simulink model "inv"  (R2024b)
settings: Solver=VariableStepAuto  StartTime=0.0  StopTime=0.5  RelTol=1e-3
InitFcn:
  | systemIni
values from neighbouring files (symbols this model uses):
  omega = 1    [systemIni.m]
  PWMrat = 39    [systemIni.m]
  Tc = 10e-6    (= 1e-05)    [systemIni.m]
  Ts = 1e-6    (= 1e-06)    [systemIni.m]
  v_ref = Vdc    [systemIni.m]
  Vdc = 550/Vb    [systemIni.m]
  w_b = wb    [systemIni.m]
libraries: spspowerguiLib x2
settings Model: Creator=PetrosK  LastModifiedBy=horak
settings DebuggingCC: UnderspecifiedInitializationDetection=Classic  MergeDetectMultiDrivingBlocksExec=none
settings ModelReferenceCC: PropagateSignalLabelsOutOfModel=off

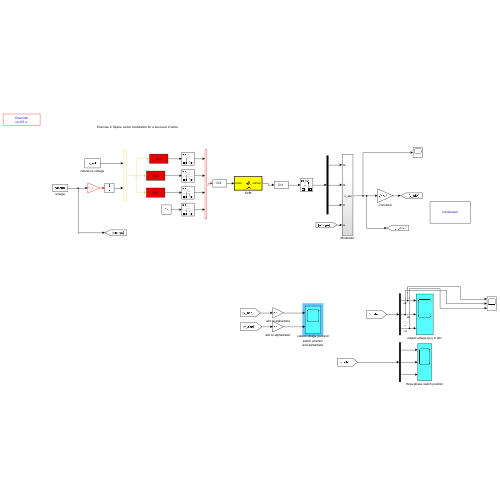
[thumbnail: Simulink's stored preview of the top-level diagram]
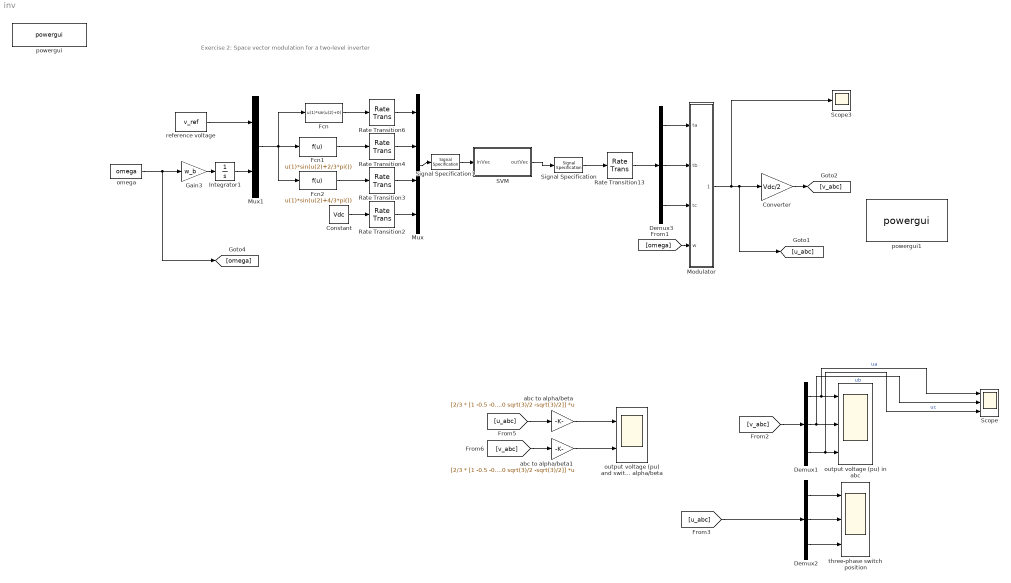
== system inv ==
  note: Exercise 2: Space vector modulation for a two-level inverter
  Constant : Constant  Value=Vdc  VectorParams1D=off
  Converter : Gain  Gain=Vdc/2  SaturateOnIntegerOverflow=on  OutDataTypeStr=Inherit: Same as input  ParamDataTypeStr=Inherit: Same as input
  Demux1 : Demux  Outputs=3
  Demux2 : Demux  Outputs=3
  Demux3 : Demux  Outputs=3
  Fcn : Fcn  Expr=u(1)*sin(u(2)+0)
  Fcn1 : Fcn  Expr=u(1)*sin(u(2)+2/3*pi())
  Fcn2 : Fcn  Expr=u(1)*sin(u(2)+4/3*pi())
  Gain3 : Gain  Gain=w_b
  Integrator1 : Integrator
  Modulator : Subsystem
  Mux : Mux
  Mux1 : Mux  Inputs=2
  Rate Transition13 : RateTransition  Deterministic=off  OutPortSampleTime=Ts
  Rate Transition{2..4,6} (4 alike) : RateTransition  Deterministic=off  OutPortSampleTime=Tc
  SVM : MATLAB Function  TreatAsAtomicUnit=on
  Scope : Scope  NumInputPorts=3
  Scope3 : Scope
  Signal Specification : SignalSpecification  Dimensions=3
  Signal Specification1 : SignalSpecification  Dimensions=4
  abc to alpha/beta : Gain  Gain=[2/3 * [1 -0.5 -0.5;0 sqrt(3)/2 -sqrt(3)/2]]  Multiplication=Matrix(K*u)  SaturateOnIntegerOverflow=on  OutDataTypeStr=Inherit: Same as input  ParamDataTypeStr=Inherit: Same as input
  abc to alpha/beta1 : Gain  Gain=[2/3 * [1 -0.5 -0.5;0 sqrt(3)/2 -sqrt(3)/2]]  Multiplication=Matrix(K*u)  SaturateOnIntegerOverflow=on  OutDataTypeStr=Inherit: Same as input  ParamDataTypeStr=Inherit: Same as input
  omega : Constant  Value=omega  VectorParams1D=off
  output voltage (pu) and switch position and alpha/beta : Scope  NumInputPorts=2
  output voltage (pu) in abc : Scope  NumInputPorts=3
  powergui : spspowerguiLib/powergui  Priority=1  SimulationMode=Discrete  SampleTime=Tc  frequency=60  Iterations=50  frequencyindice=0  Pbase=100e6  ErrMax=1e-4  UnitsV=kV  UnitsW=MW  buscounter=0  FunctionMessages=off  echomessages=off  EnableUseOfTLC=off  CurrentSourceSwitches=off  DisableSnubberDevices=off  DisableRonSwitches=off  DisableVfSwitches=off  DisplayEquations=off  AutomaticDiscreteSolvers=off  SolverType=Tustin  Interpol=off  ExternalGateDelay=off  methode=off  Ts=0  x0status=zero  SPID=off  SwTol=0  HookPort=off  NonlinearTolerance=1e-4  nMaxIteration=100  ContinueOnMaxIteration=off  RestoreLinks=warning  ResistiveCurrentMeasurement=off  Frange=[0:2:500]  Ylog=off  Xlog=on  ShowGrid=off  save=off  variable=ZData  structure=u_alpha  ZoomFFT=off  StartTime=0.02  cycles=1  DisplayStyle=1  fundamental=50  FreqAxis=off  MaxFrequency=4000  frequencyindicesteady=1  RmsSteady=1  display=off
  powergui1 : spspowerguiLib/powergui  Priority=1  SimulationMode=Continuous  SampleTime=50e-6  frequency=60  Iterations=50  frequencyindice=60  Pbase=100e6  ErrMax=1e-4  UnitsV=kV  UnitsW=MW  buscounter=0  FunctionMessages=off  echomessages=on  EnableUseOfTLC=off  CurrentSourceSwitches=off  DisableSnubberDevices=off  DisableRonSwitches=off  DisableVfSwitches=off  DisplayEquations=off  AutomaticDiscreteSolvers=off  SolverType=Tustin/Backward Euler (TBE)  Interpol=off  ExternalGateDelay=off  methode=off  Ts=100  x0status=blocks  SPID=on  SwTol=0  HookPort=off  NonlinearTolerance=1e-4  nMaxIteration=100  ContinueOnMaxIteration=off  RestoreLinks=warning  ResistiveCurrentMeasurement=off  Frange=[0:2:500]  Ylog=off  Xlog=on  ShowGrid=off  save=off  variable=ZData  structure=0  ZoomFFT=off  StartTime=0.0  cycles=1  DisplayStyle=1  fundamental=60  FreqAxis=off  MaxFrequency=1000  frequencyindicesteady=1  RmsSteady=1  display=off
  reference voltage : Constant  Value=v_ref  VectorParams1D=off
  three-phase switch position : Scope  NumInputPorts=3
  wires:
  SVM/1(outVec) -> Signal Specification/1
  Demux3/2 -> Modulator/2(tb)
  Demux3/3 -> Modulator/3(tc)
  Demux3/1 -> Modulator/1(ta)
  Constant/1 -> Rate Transition2/1
  Rate Transition13/1 -> Demux3/1
  Signal Specification1/1 -> SVM/1(inVec)
  Signal Specification/1 -> Rate Transition13/1
  Mux/1 -> Signal Specification1/1
  Rate Transition2/1 -> Mux/4
  Rate Transition3/1 -> Mux/3
  Rate Transition4/1 -> Mux/2
  Rate Transition6/1 -> Mux/1
  Fcn/1 -> Rate Transition6/1
  Fcn1/1 -> Rate Transition4/1
  Fcn2/1 -> Rate Transition3/1
  Mux1/1 -> Fcn2/1, Fcn1/1, Fcn/1
  [omega] -> Modulator/4(w)
  reference voltage/1 -> Mux1/1
  Gain3/1 -> Integrator1/1
  Integrator1/1 -> Mux1/2
  Demux1/2 -> Scope/2, output voltage (pu) in abc/2  "ub"
  Demux1/3 -> Scope/3, output voltage (pu) in abc/3  "uc"
  abc to alpha/beta/1 -> output voltage (pu) and switch position and alpha/beta/1
  [v_abc] -> Demux1/1
  abc to alpha/beta1/1 -> output voltage (pu) and switch position and alpha/beta/2
  [u_abc] -> abc to alpha/beta/1
  [v_abc] -> abc to alpha/beta1/1
  Modulator/1(u_abc) -> Scope3/1, [u_abc], Converter/1
  omega/1 -> [omega], Gain3/1
  Demux1/1 -> Scope/1, output voltage (pu) in abc/1  "ua"
  Demux2/2 -> three-phase switch position/2
  [u_abc] -> Demux2/1
  Demux2/1 -> three-phase switch position/1
  Demux2/3 -> three-phase switch position/3
  Converter/1 -> [v_abc]

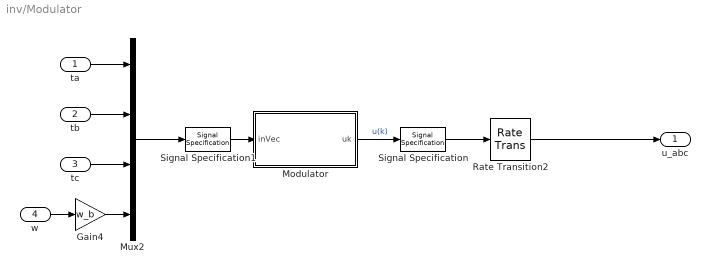
== system inv/Modulator ==
  ta : Inport
  tb : Inport  Port=2
  tc : Inport  Port=3
  w : Inport  Port=4
  Gain4 : Gain  Gain=w_b
  Modulator : MATLAB Function  TreatAsAtomicUnit=on
  Mux2 : Mux
  Rate Transition2 : RateTransition  OutPortSampleTime=Ts
  Signal Specification : SignalSpecification  Dimensions=3
  Signal Specification1 : SignalSpecification  Dimensions=4
  u_abc : Outport
  wires:
  ta/1 -> Mux2/1
  tb/1 -> Mux2/2
  tc/1 -> Mux2/3
  Modulator/1(uk) -> Signal Specification/1  "u(k)"
  Signal Specification/1 -> Rate Transition2/1
  Rate Transition2/1 -> u_abc/1
  Mux2/1 -> Signal Specification1/1
  w/1 -> Gain4/1
  Signal Specification1/1 -> Modulator/1(inVec)
  Gain4/1 -> Mux2/4

== matlab function inv/Modulator/Modulator ==
  data: inVec input; uk output; PWMrat parameter; Ts parameter
function uk = modulator(inVec, PWMrat, Ts)

% generation of switching signals for a three-phase two-level inverter
%
% Control of Electrical Drive Systems, TAU, Tampere
% Petros Karamanakos, September 2025

persistent kk carrier
persistent t

% interface
t_a = 2 * inVec(1) - 1; % modulating signal of phase a in [-1, 1]
t_b = 2 * inVec(2) - 1;	% modulating signal of phase b in [-1, 1]
t_c = 2 * inVec(3) - 1; % modulating signal of phase c in [-1, 1]
w  = inVec(4);          % angular speed [pu]

 t = [t_a; t_b; t_c];


if isempty(kk)
    kk = 1;
    carrier = 0;
    t = [t_a; t_b; t_c];
end

% fundamental frequency/period
f_1 = w/(2 * pi);
T_1 = 1/f_1;

% period of carrier
TsPWM =  T_1/PWMrat ;% to be added

if kk * Ts < TsPWM
    triangleStep = Ts/TsPWM *4; % to be added
    if kk*Ts <= TsPWM/4
        carrier = carrier - triangleStep;
    elseif kk*Ts > TsPWM/4 &&  kk*Ts <= 3*TsPWM/4
        carrier = carrier + triangleStep;
    else
        
        carrier = carrier - triangleStep;
    end
else 
    kk = 0;
    carrier = 0;
end
% if(1-abs(carrier)<triangleStep)
%         t = [t_a; t_b; t_c];
% end
kk = kk + 1;

%% asymmetric regular sampling
% to be added
tmp=t>(carrier*ones(3,1));
uk=tmp*2-1;
%% generate the switching signals
 % to be added

%% output signal

% uk = [u_a; u_b; u_c];   % three-phase switch position

return

== matlab function inv/SVM ==
  data: inVec input; outVec output
function outVec  = SVM(inVec)

% SVM for a three-phase two-level inverter
%
% Control of Electrical Drive Systems, TAU, Tampere
% Petros Karamanakos, September 2025

v_a = inVec(1);
v_b = inVec(2);
v_c = inVec(3);
Vdc = inVec(4);

v_abc = [v_a; v_b; v_c];

% reduced Clarke transformation
K = 2/3 * [1 -0.5 -0.5;           	% abc -> alpha/beta
           0 sqrt(3)/2 -sqrt(3)/2];     
           
%% SVM --> to be added

% derive the modulating signal in alpha/beta
v_ab=K*v_abc;

% identify the sector the modulating signal is located
[th_neg,u_nor]=cart2pol(v_ab(1),v_ab(2));
th=mod(th_neg,2*pi());
ang=0:2/6*pi():2*pi();

m=u_nor/Vdc;%% todo !!!!!!!!!!!!!!!!
[~,sector]=find(ang<th,1,"last");
f1=ang(sector);
f2=ang(sector+1);

sectorr=sector(1);

Dti=det([m*cos(th-f1),u_nor*cos(pi()/3); ...
     m*cos(f2-th) , u_nor]);
Dtj=det([u_nor, m*cos(th-f1);...
    u_nor*cos(pi()/3), m*cos(f2-th)]);
D=u_nor^2*(1-cos(pi()/3)^2);

ta=Dti/D; %i
tb=Dtj/D; %j
tc=1-ta-tb; %k
ti=[ta;tb;tc];
% compute 
%   ta --> application time of voltage vector v_i 
%   tb --> application time of voltage vector v_j
%   t0 --> application time of zero vectors
% based on Cramer's rule
sectors=cat(3,[1 1 1/2; 0 1 1/2; 0 0 1/2],[1 0 1/2; 1 1 1/2; 0 0 1/2],[0 0 1/2; 1 1 1/2; 0 1 1/2],...
              [0 0 1/2; 1 0 1/2; 1 1 1/2],[0 1 1/2; 0 0 1/2; 1 1 1/2],[1 1 1/2; 0 0 1/2; 1 0 1/2]);
% tmp=zeros(3,1)
tmp=sectors(:,:,sector)*[ta;tb;tc];

% calculation of application times based on sectors
%   t1 --> time the upper switch in phase a is on
%   t3 --> time the upper switch in phase b is on
%   t5 --> time the upper switch in phase c is on

%% switching times for the three upper switches
% outVec = [t1; t3; t5];
outVec=[tmp(1),tmp(2),tmp(3)];
return
